simulink library "sysgenImageTileReconstructionDemoLib"  (Simulink 7.5)
settings: Solver=ode45  StartTime=0.0  StopTime=10.0  RelTol=1e-3
undefined symbols (not defined in the file or in its folder): a, b, c_image_rows, c_num_fstores, c_swathe_size
libraries: xbsIndex_r4 x22, sysgenImageTileReconstructionDemoLib x1
settings Model: Creator=arvinds  LastModifiedBy=arvinds

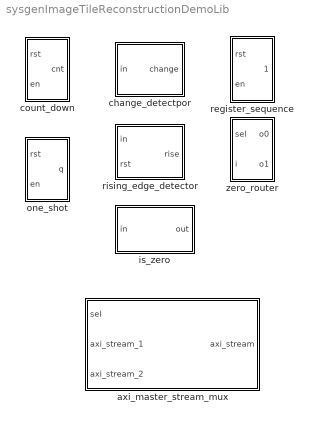
== system sysgenImageTileReconstructionDemoLib ==
  axi_master_stream_mux : Subsystem
  change_detectpor : Subsystem
  count_down : Subsystem  mask{init_val=16}
      mask prompts: init_val "Initial Value"
  is_zero : Subsystem
      mask Display: disp('==0')
  one_shot : Subsystem
  register_sequence : Subsystem  mask{c_sequence=[1 0 11]}
      mask prompts: c_sequence "User sequence"
  rising_edge_detector : Subsystem
      mask Display: disp('\lceil','texmode','on')
  zero_router : Subsystem

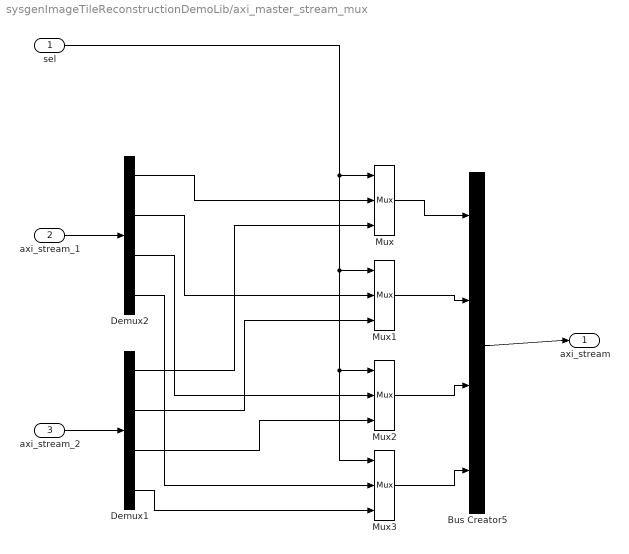
== system sysgenImageTileReconstructionDemoLib/axi_master_stream_mux ==
  sel : Inport
  axi_stream_1 : Inport  Port=2
  axi_stream_2 : Inport  Port=3
  Bus Creator5 : BusCreator
  Demux1 : Demux  BusSelectionMode=on
  Demux2 : Demux  BusSelectionMode=on
  Mux{,1..3} (4 alike) : xbsIndex_r4/Mux  inputs=2  en=off  latency=0  precision=Full  arith_type=Unsigned  n_bits=16  bin_pt=14  quantization=Truncate  overflow=Wrap  dbl_ovrd=off  block_type=mux
      settings: block_version=12.3
  axi_stream : Outport
  wires:
  axi_stream_1/1 -> Demux2/1
  axi_stream_2/1 -> Demux1/1
  sel/1 -> Mux3/1, Mux2/1, Mux1/1, Mux/1
  Demux2/1 -> Mux/2
  Demux2/2 -> Mux1/2
  Demux2/3 -> Mux2/2
  Demux2/4 -> Mux3/2
  Demux1/1 -> Mux/3
  Demux1/2 -> Mux1/3
  Demux1/3 -> Mux2/3
  Demux1/4 -> Mux3/3
  Mux/1 -> Bus Creator5/1
  Mux1/1 -> Bus Creator5/2
  Mux2/1 -> Bus Creator5/3
  Mux3/1 -> Bus Creator5/4
  Bus Creator5/1 -> axi_stream/1

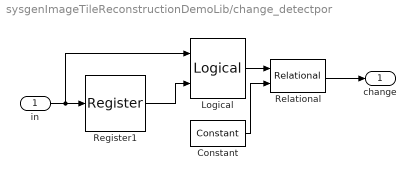
== system sysgenImageTileReconstructionDemoLib/change_detectpor ==
  in : Inport
  Constant : xbsIndex_r4/Constant  arith_type=Unsigned  const=0  n_bits=1  bin_pt=0  explicit_period=off  period=1  equ=P=C  opselect=C  inp2=PCIN>>17  opr=+  inp1=P  carry=CIN  dbl_ovrd=off  block_type=constant
      settings: block_version=12.3
  Logical : xbsIndex_r4/Logical  logical_function=XOR  inputs=2  en=off  latency=0  precision=Full  arith_type=Unsigned  n_bits=16  bin_pt=0  align_bp=on  dbl_ovrd=off  block_type=logical
      settings: block_version=12.3
  Register1 : xbsIndex_r4/Register  init=0  rst=off  en=off  dbl_ovrd=off  block_type=register
      settings: block_version=12.3
  Relational : xbsIndex_r4/Relational  mode=a!=b  en=off  latency=0  dbl_ovrd=off  block_type=relational
      settings: block_version=12.3
  change : Outport
  wires:
  Register1/1 -> Logical/2
  in/1 -> Register1/1, Logical/1
  Logical/1 -> Relational/1
  Constant/1 -> Relational/2
  Relational/1 -> change/1

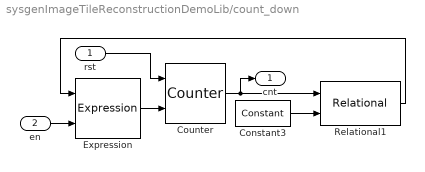
== system sysgenImageTileReconstructionDemoLib/count_down ==
  rst : Inport
  en : Inport  Port=2
  Constant3 : xbsIndex_r4/Constant  arith_type=Unsigned  const=0  n_bits=ceil(ceil( (c_image_rows/c_swathe_size) / c_num_fstores) + 1)  bin_pt=0  explicit_period=off  period=1  equ=P=C  opselect=C  inp2=PCIN>>17  opr=+  inp1=P  carry=CIN  dbl_ovrd=off  block_type=constant
      settings: block_version=12.3
  Counter : xbsIndex_r4/Counter  cnt_type=Count Limited  cnt_to=0  operation=Down  start_count=init_val  cnt_by_val=1  arith_type=Unsigned  n_bits=ceil(log2(init_val + 1))  bin_pt=0  load_pin=off  rst=on  en=on  explicit_period=on  period=1  dbl_ovrd=off  use_behavioral_HDL=off  implementation=Fabric  block_type=counter
      settings: block_version=12.3
  Expression : xbsIndex_r4/Expression  expression=a & b  align_bp=on  en=off  latency=0  precision=Full  arith_type=Unsigned  n_bits=16  bin_pt=0  dbl_ovrd=off  block_type=expr
      settings: block_version=12.3
  Relational1 : xbsIndex_r4/Relational  mode=a!=b  en=off  latency=0  dbl_ovrd=off  block_type=relational
      settings: block_version=12.3
  cnt : Outport  OutDataType=fixdt(1, 16)  OutScaling=2^0
  wires:
  en/1 -> Expression/2
  Relational1/1 -> Expression/1
  Constant3/1 -> Relational1/2
  Counter/1 -> cnt/1, Relational1/1
  Expression/1 -> Counter/2
  rst/1 -> Counter/1

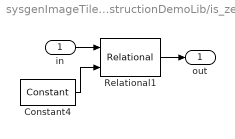
== system sysgenImageTileReconstructionDemoLib/is_zero ==
  in : Inport
  Constant4 : xbsIndex_r4/Constant  arith_type=Unsigned  const=0  n_bits=1  bin_pt=0  explicit_period=off  period=1  equ=P=C  opselect=C  inp2=PCIN>>17  opr=+  inp1=P  carry=CIN  dbl_ovrd=off  block_type=constant
      settings: block_version=12.3
  Relational1 : xbsIndex_r4/Relational  mode=a=b  en=off  latency=0  dbl_ovrd=off  block_type=relational
      settings: block_version=12.3
  out : Outport
  wires:
  Constant4/1 -> Relational1/2
  in/1 -> Relational1/1
  Relational1/1 -> out/1

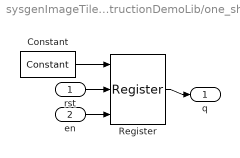
== system sysgenImageTileReconstructionDemoLib/one_shot ==
  rst : Inport
  en : Inport  Port=2
  Constant : xbsIndex_r4/Constant  arith_type=Boolean  const=1  n_bits=16  bin_pt=14  explicit_period=off  period=1  equ=P=C  opselect=C  inp2=PCIN>>17  opr=+  inp1=P  carry=CIN  dbl_ovrd=off  block_type=constant
      settings: block_version=12.3
  Register : xbsIndex_r4/Register  init=0  rst=on  en=on  dbl_ovrd=off  block_type=register
      settings: block_version=12.3
  q : Outport
  wires:
  Constant/1 -> Register/1
  rst/1 -> Register/2
  Register/1 -> q/1
  en/1 -> Register/3

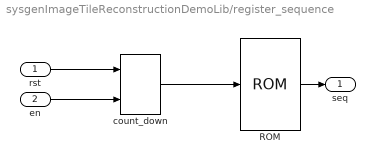
== system sysgenImageTileReconstructionDemoLib/register_sequence ==
  rst : Inport
  en : Inport  Port=2
  ROM : xbsIndex_r4/ROM  depth=length(c_sequence)  initVector=c_sequence  distributed_mem=Distributed memory  rst=off  init_reg=0  en=off  latency=0  arith_type=Unsigned  n_bits=32  bin_pt=0  dbl_ovrd=off  optimize=Area  use_rpm=on  block_type=sprom
      settings: block_version=12.3
  count_down : sysgenImageTileReconstructionDemoLib/count_down  SystemSampleTime=-1  init_val=length(c_sequence)-1
  seq : Outport
  wires:
  count_down/1 -> ROM/1
  rst/1 -> count_down/1
  ROM/1 -> seq/1
  en/1 -> count_down/2

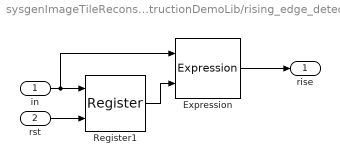
== system sysgenImageTileReconstructionDemoLib/rising_edge_detector ==
  in : Inport
  rst : Inport  Port=2
  Expression : xbsIndex_r4/Expression  expression=a & ~b  align_bp=on  en=off  latency=0  precision=Full  arith_type=Unsigned  n_bits=16  bin_pt=0  dbl_ovrd=off  block_type=expr
      settings: block_version=12.3
  Register1 : xbsIndex_r4/Register  init=0  rst=on  en=off  dbl_ovrd=off  block_type=register
      settings: block_version=12.3
  rise : Outport
  wires:
  Expression/1 -> rise/1
  in/1 -> Register1/1, Expression/1
  Register1/1 -> Expression/2
  rst/1 -> Register1/2

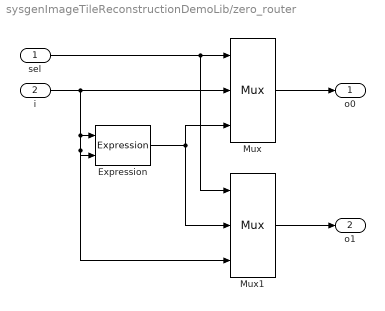
== system sysgenImageTileReconstructionDemoLib/zero_router ==
  sel : Inport  OutDataType=fixdt(1, 16)  OutScaling=2^0
  i : Inport  Port=2  OutDataType=fixdt(1, 16)  OutScaling=2^0
  Expression : xbsIndex_r4/Expression  expression=a ^ b  align_bp=on  en=off  latency=0  precision=Full  arith_type=Unsigned  n_bits=16  bin_pt=0  dbl_ovrd=off  block_type=expr
      settings: block_version=12.3
  Mux : xbsIndex_r4/Mux  inputs=2  en=off  latency=0  precision=Full  arith_type=Unsigned  n_bits=16  bin_pt=14  quantization=Truncate  overflow=Wrap  dbl_ovrd=off  block_type=mux
      settings: block_version=12.3
  Mux1 : xbsIndex_r4/Mux  inputs=2  en=off  latency=0  precision=Full  arith_type=Unsigned  n_bits=16  bin_pt=14  quantization=Truncate  overflow=Wrap  dbl_ovrd=off  block_type=mux
      settings: block_version=12.3
  o0 : Outport  OutDataType=fixdt(1, 16)  OutScaling=2^0
  o1 : Outport  Port=2  OutDataType=fixdt(1, 16)  OutScaling=2^0
  wires:
  Expression/1 -> Mux/3, Mux1/2
  sel/1 -> Mux/1, Mux1/1
  i/1 -> Mux/2, Expression/1, Expression/2, Mux1/3
  Mux/1 -> o0/1
  Mux1/1 -> o1/1
